simulink model "adc_preproc_core"  (R2012b)
settings: Solver=VariableStepDiscrete  SolverMode=SingleTasking  StartTime=0.0  StopTime=40960  RelTol=1e-3
undefined symbols (not defined in the file or in its folder): A, B, fixpnt, PCIN, xlipgetpartsetting
libraries: xbsIndex_r4 x537, casper_library_sources x8, casper_library_misc x8, simulink x1
(part 9 of 9)

== system adc_preproc_core/adc_preproc_core/noise_gen0/noise7/wgn/u2n/cosin_vanilla ==
  theta : Inport
  Delay : xbsIndex_r4/Delay  rst=off  infoeditControl=Selection of Reset will increase slice count due to use of real FFs and instead of SRLs  en=off  latency=bram_latency  dbl_ovrd=off  reg_retiming=on  block_type=delay
  ROM : xbsIndex_r4/ROM  depth=2^(11)  initVector=[127 127 383 383 639 639 639 895 895 1151 1151 1151 1407 1407 1407 1663 1663 1919 1919 1919 2175 2175 2431 2431 2431 2687 2687 2943 2943 2943 3199 3199 3455 3455 3455 3711 3711 3711 3967 3967 4223 4223 4223 4479 4479 4735 4735 4735 4991 4991 5246 5246 5246 5502 5502 5502 5758 5758 6014 6014 6014 6270 6270 6526 6526 6525 6781 6781 7037 7037 7037 7293 7293 7293 7549 7549 7805 7804 7804 8060 8060 8060 8316 8316 8572 8572 8572 8827 8827 9083 9083 9083 9339 9339 9339 9595 9594 9850 9850 9850 10106 10106 10106 10362 10362 10617 10617 10617 10873 10873 10873 11129 11129 11128 11384 11384 11640 11640 11640 11896 11895 11895 12151 12151 12407 12407 12407 12662 12662 12662 12918 12918 12918 13173 13173 13429 13429 13429 13685 13685 13684 13940 13940 13940 14196 14196 14195 14451 14451 14451 14707 14707 14962 14962 14962 15218 15218 15217 15473 15473 15473 15729 15729 15728 15984 15984 15984 16240 16239 16239 16495 16495 16495 16750 16750 16750 17006 17006 17005 17261 17261 17261 17517 17516 17516 17772 17772 17772 18027 18027 18027 18283 18282 18282 18538 18538 18538 18793 18793 18793 19049 19048 19048 19304 19304 19304 19559 19559 19559 19815 19814 19814 20070 20070 20069 20069 20325 20325 20324 20580 20580 20580 20835 20835 20835 21091 21090 21090 21090 21346 21345 21345 21601 21601 21600 21600 21856 21856 21855 22111 22111 22111 22366 22366 22366 22366 22621 22621 22621 22876 22876 22876 22876 23131 23131 23131 23387 23386 23386 23386 23641 23641 23641 23641 23896 23896 23896 24151 24151 24151 24151 24406 24406 24406 24405 24661 24661 24660 24660 24916 24916 24915 24915 25171 25170 25170 25170 25426 25425 25425 25425 25680 25680 25680 25679 25935 25935 25934 25934 26190 26190 26189 26189 26445 26444 26444 26444 26699 26699 26699 26698 26698 26954 26953 26953 26953 27208 27208 27208 27207 27207 27463 27462 27462 27462 27717 27717 27717 27716 27716 27972 27971 27971 27971 27970 28226 28226 28225 28225 28225 28480 28480 28480 28479 28479 28735 28734 28734 28734 28733 28989 28989 28988 28988 28988 28987 29243 29243 29242 29242 29242 29497 29497 29496 29496 29496 29495 29751 29751 29750 29750 29750 29749 30005 30005 30004 30004 30004 30003 30003 30258 30258 30258 30257 30257 30257 30512 30512 30512 30511 30511 30510 30510 30766 30765 30765 30765 30764 30764 30763 31019 31019 31018 31018 31018 31017 31017 31017 31272 31272 31271 31271 31271 31270 31270 31270 31269 31525 31524 31524 31524 31523 31523 31523 31522 31522 31777 31777 31777 31776 31776 31775 31775 31775 31774 31774 32030 32029 32029 32028 32028 32028 32027 32027 32027 32026 32026 32025 32281 32281 32280 32280 32279 32279 32279 32278 32278 32277 32277 32277 32276 32276 32276 32531 32531 32530 32530 32530 32529 32529 32528 32528 32528 32527 32527 32526 32526 32526 32525 32525 32525 32524 32524 32523 32523 32523 32522 32522 32521 32521 32521 32520 32520 32519 32519 32519 32518 32518 32517 32517 32517 32516 32516 32516 32515 32515 32514 32514 32514 32513 32513 32512 32512 32512 32767 32767 32766 32766 32766 32765 32765 32764 32764 32764 32763 32763 32763 32762 32762 32761 32761 32761 32760 32760 32759 32759 32759 32758 32758 32757 32757 32757 32756 32756 32755 32755 32755 32754 32754 32754 32753 32753 32752 32752 32752 32751 32751 32750 32750 32750 32749 32749 32492 32492 32492 32491 32491 32491 32490 32490 32489 32489 32489 32488 32488 32487 32487 32231 32230 32230 32229 32229 32229 32228 32228 32228 32227 32227 32226 31970 31970 31969 31969 31969 31968 31968 31967 31967 31967 31710 31710 31709 31709 31709 31708 31708 31708 31707 31451 31450 31450 31450 31449 31449 31449 31448 31448 31191 31191 31191 31190 31190 31190 31189 31189 30933 30932 30932 30931 30931 30931 30930 30674 30674 30673 30673 30672 30672 30672 30415 30415 30415 30414 30414 30414 30157 30157 30156 30156 30156 30155 30155 29899 29898 29898 29898 29897 29897 29641 29640 29640 29640 29639 29639 29382 29382 29382 29381 29381 29125 29124 29124 29124 29123 29123 28867 28866 28866 28866 28865 28609 28609 28608 28608 ...(+8071 chars)]  distributed_mem=Block RAM  rst=off  init_reg=0  en=off  latency=bram_latency  gui_display_data_type=Fixed-point  arith_type=Unsigned  n_bits=n_bits*2  bin_pt=0  preci_type=Single  exp_width=8  frac_width=24  dbl_ovrd=off  optimize=Speed  use_rpm=on  block_type=sprom
  assert : xbsIndex_r4/Assert  assert_type=on  type_source=Explicitly  gui_display_data_type=Fixed-point  arith_type=Unsigned  n_bits=11  bin_pt=0  preci_type=Single  exp_width=8  frac_width=24  assert_rate=off  rate_source=Explicitly  period=1  output_port=on  block_type=assert
  c_to_ri : casper_library_misc/c_to_ri  n_bits=n_bits  bin_pt=bin_pt
      settings: AttributesFormatString=8_7 r/i
  misci : xbsIndex_r4/Constant  const=0  gui_display_data_type=Fixed-point  arith_type=Unsigned  n_bits=1  bin_pt=0  preci_type=Single  exp_width=8  frac_width=24  explicit_period=on  period=1  equ=P=C  opselect=C  inp2=PCIN>>17  opr=+  inp1=P  carry=CIN  dbl_ovrd=off  block_type=constant
  misco : Terminator
  sin : Outport
  cos : Outport  Port=2
  wires:
  theta/1 -> assert/1
  assert/1 -> ROM/1
  ROM/1 -> c_to_ri/1
  c_to_ri/1 -> sin/1
  c_to_ri/2 -> cos/1
  misci/1 -> Delay/1
  Delay/1 -> misco/1
